simulink model "Exmaple_P1"  (R2017b)
settings: Solver=VariableStepAuto  StartTime=0.0  StopTime=inf  RelTol=1e-3
libraries: Project1_Library x3, simulink x2, realtime_pacer_lib x1
settings Model: Creator=hattanbadyah  LastModifiedBy=hattanbadyah

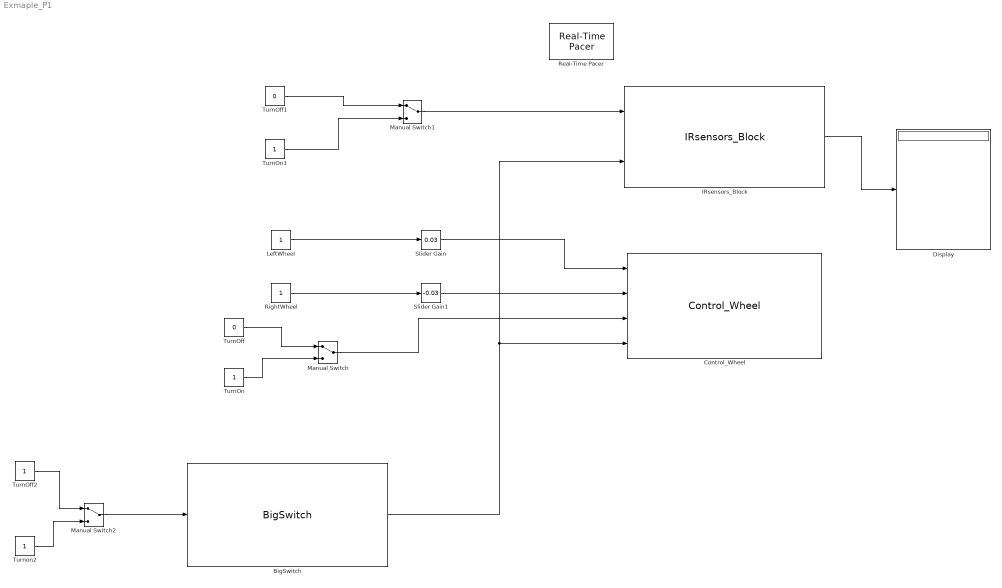
== system Exmaple_P1 ==
  BigSwitch : Project1_Library/BigSwitch
  Control_Wheel : Project1_Library/Control_Wheel
  Display : Display
  IRsensors_Block : Project1_Library/IRsensors_Block
  LeftWheel : Constant
  Manual Switch : ManualSwitch
  Manual Switch1 : ManualSwitch
  Manual Switch2 : ManualSwitch
  Real-Time Pacer : realtime_pacer_lib/Real-Time Pacer  simTimePerRealTime=1
  RightWheel : Constant
  Slider Gain : simulink/Math Operations/Slider Gain  gain=0.03  low=-0.5  high=0.5
  Slider Gain1 : simulink/Math Operations/Slider Gain  gain=-0.03  low=-0.5  high=0.5
  TurnOff : Constant  Value=0
  TurnOff1 : Constant  Value=0
  TurnOff2 : Constant
  TurnOn : Constant
  TurnOn1 : Constant
  Turnon2 : Constant
  wires:
  BigSwitch/1 -> IRsensors_Block/2, Control_Wheel/4
  RightWheel/1 -> Slider Gain1/1
  LeftWheel/1 -> Slider Gain/1
  Slider Gain/1 -> Control_Wheel/1
  Slider Gain1/1 -> Control_Wheel/2
  TurnOff/1 -> Manual Switch/1
  TurnOn/1 -> Manual Switch/2
  Manual Switch/1 -> Control_Wheel/3
  Manual Switch1/1 -> IRsensors_Block/1
  TurnOff1/1 -> Manual Switch1/1
  TurnOn1/1 -> Manual Switch1/2
  IRsensors_Block/1 -> Display/1
  Manual Switch2/1 -> BigSwitch/1
  TurnOff2/1 -> Manual Switch2/1
  Turnon2/1 -> Manual Switch2/2
